simulink model "Question_17"  (R2022b)
settings: Solver=VariableStepAuto  StartTime=0.0  StopTime=20.0  RelTol=1e-3
settings Model: Creator=adlercohen  LastModifiedBy=adlercohen

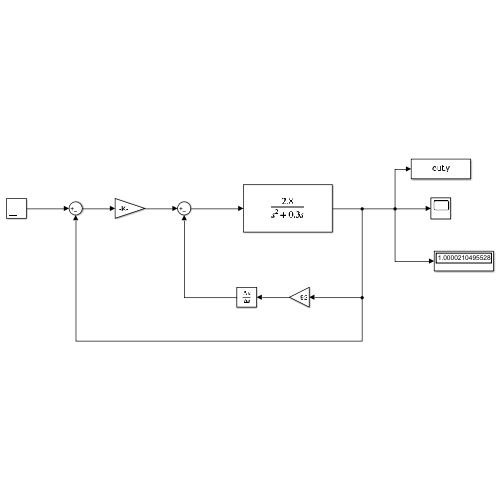
[thumbnail: Simulink's stored preview of the top-level diagram]
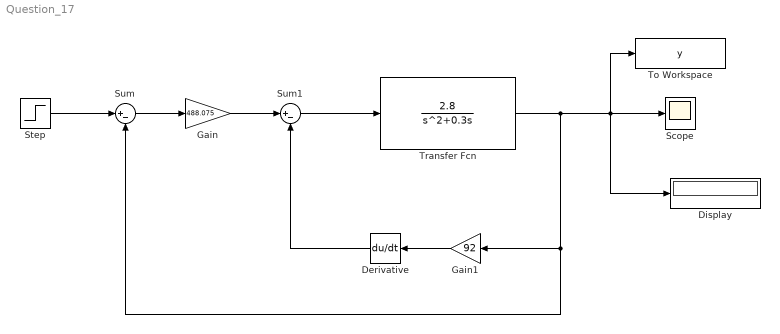
== system Question_17 ==
  Derivative : Derivative
  Display : Display
  Gain : Gain  Gain=488.075
  Gain1 : Gain  Gain=92
  Scope : Scope
  Step : Step  Time=0  SampleTime=0
  Sum : Sum  Inputs=|+-
  Sum1 : Sum  Inputs=|+-
  To Workspace : ToWorkspace  VariableName=y  SampleTime=-1
  Transfer Fcn : TransferFcn  Numerator=[2.8]  Denominator=[1 0.3 0]
  wires:
  Step/1 -> Sum/1
  Sum/1 -> Gain/1
  Gain/1 -> Sum1/1
  Sum1/1 -> Transfer Fcn/1
  Transfer Fcn/1 -> Gain1/1, Sum/2, To Workspace/1, Display/1, Scope/1
  Gain1/1 -> Derivative/1
  Derivative/1 -> Sum1/2
